simulink model "VdP_RCAC_ESC_sim"  (R2023b)
settings: Solver=ode4  StartTime=0.0  StopTime=Tf  FixedStep=Ts  RelTol=1e-3
values from neighbouring files (symbols this model uses):
  T_samp = 10    [VdP_RCAC_ESC.m]
  t_start = 20    [VdP_CL.m]    (also in VdP_RCAC_ESC.m)
  Ts = 0.001    [VdP_CL.m]    (also in VdP_RCAC_ESC.m)
  x0 = [1;0]    [VdP_CL.m]    (also in VdP_RCAC_ESC.m)
libraries: dspstat3 x1, matrix_library x1
settings Model: Creator=Juan Augusto Paredes  LastModifiedBy=Juan Augusto Paredes

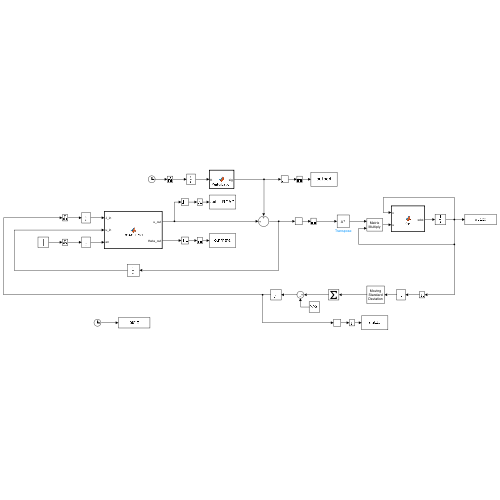
[thumbnail: Simulink's stored preview of the top-level diagram]
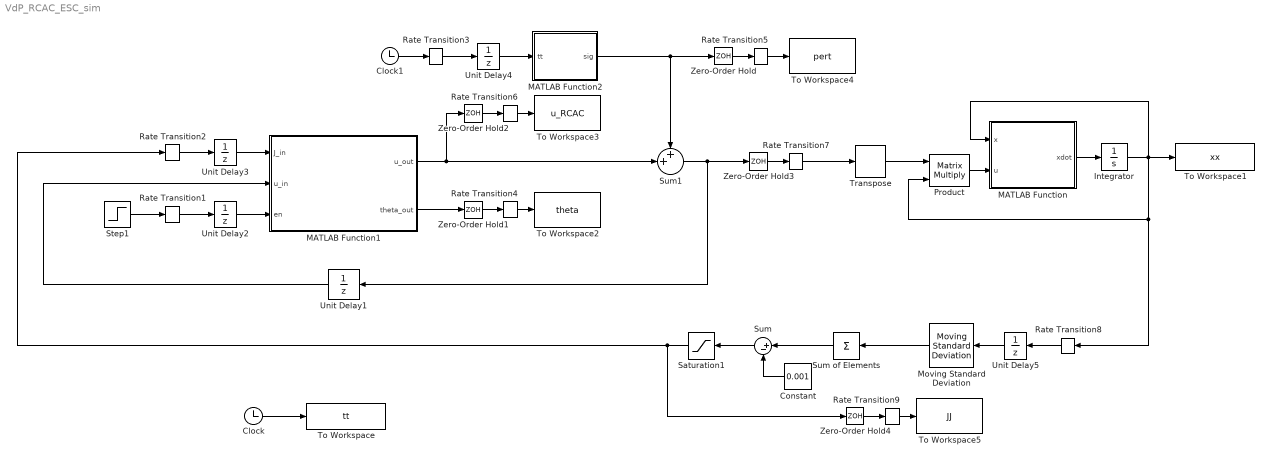
== system VdP_RCAC_ESC_sim ==
  Clock : Clock
  Clock1 : Clock
  Constant : Constant  Value=0.001
  Integrator : Integrator  InitialCondition=x0
  MATLAB Function : MATLAB Function  TreatAsAtomicUnit=on
  MATLAB Function1 : MATLAB Function  TreatAsAtomicUnit=on
  MATLAB Function2 : MATLAB Function  TreatAsAtomicUnit=on
  Moving Standard Deviation : dspstat3/Moving Standard Deviation  Method=Sliding window  ForgettingFactorPort=off  SpecifyWindowLength=on  WindowLength=5000  OverlapLength=4999  AllowArbitraryInputLength=off  ForgettingFactor=0.9  SimulateUsing=Code generation
  Product : Product  Multiplication=Matrix(*)
  Rate Transition{1..4,8..9} (6 alike) : RateTransition
  Rate Transition5 : RateTransition  InitialCondition=[0;0]
  Rate Transition6 : RateTransition  InitialCondition=[0;0]
  Rate Transition7 : RateTransition  InitialCondition=[0;0]
  Saturation1 : Saturate  UpperLimit=1000  LowerLimit=0
  Step1 : Step  Time=t_start  SampleTime=0
  Sum : Sum  Inputs=|+-
  Sum of Elements : Sum  Inputs=+
  Sum1 : Sum  Inputs=++|
  To Workspace : ToWorkspace  VariableName=tt  SampleTime=-1
  To Workspace1 : ToWorkspace  VariableName=xx  SampleTime=-1
  To Workspace2 : ToWorkspace  VariableName=theta  SampleTime=-1
  To Workspace3 : ToWorkspace  VariableName=u_RCAC  SampleTime=-1
  To Workspace4 : ToWorkspace  VariableName=pert  SampleTime=-1
  To Workspace5 : ToWorkspace  VariableName=JJ  SampleTime=-1
  Transpose : matrix_library/Transpose
  Unit Delay1 : UnitDelay  InitialCondition=[0;0]  SampleTime=T_samp  HasFrameUpgradeWarning=on
  Unit Delay2 : UnitDelay  SampleTime=T_samp  HasFrameUpgradeWarning=on
  Unit Delay3 : UnitDelay  SampleTime=T_samp  HasFrameUpgradeWarning=on
  Unit Delay4 : UnitDelay  SampleTime=T_samp  HasFrameUpgradeWarning=on
  Unit Delay5 : UnitDelay  SampleTime=Ts  HasFrameUpgradeWarning=on
  Zero-Order Hold{,1..4} (5 alike) : ZeroOrderHold  SampleTime=T_samp
  wires:
  MATLAB Function/1(xdot) -> Integrator/1
  Integrator/1 -> Rate Transition8/1, Product/2, To Workspace1/1, MATLAB Function/1(x)
  Clock/1 -> To Workspace/1
  Sum1/1 -> Zero-Order Hold3/1, Unit Delay1/1
  Unit Delay1/1 -> MATLAB Function1/2(u_in)
  MATLAB Function1/1(u_out) -> Zero-Order Hold2/1, Sum1/2
  Product/1 -> MATLAB Function/2(u)
  Transpose/1 -> Product/1
  Rate Transition1/1 -> Unit Delay2/1
  Unit Delay2/1 -> MATLAB Function1/3(en)
  Step1/1 -> Rate Transition1/1
  Unit Delay3/1 -> MATLAB Function1/1(J_in)
  Rate Transition2/1 -> Unit Delay3/1
  Rate Transition3/1 -> Unit Delay4/1
  Clock1/1 -> Rate Transition3/1
  Unit Delay4/1 -> MATLAB Function2/1(tt)
  Zero-Order Hold1/1 -> Rate Transition4/1
  Rate Transition4/1 -> To Workspace2/1
  MATLAB Function1/2(theta_out) -> Zero-Order Hold1/1
  MATLAB Function2/1(sig) -> Zero-Order Hold/1, Sum1/1
  Zero-Order Hold/1 -> Rate Transition5/1
  Rate Transition5/1 -> To Workspace4/1
  Zero-Order Hold2/1 -> Rate Transition6/1
  Rate Transition6/1 -> To Workspace3/1
  Zero-Order Hold3/1 -> Rate Transition7/1
  Rate Transition7/1 -> Transpose/1
  Moving Standard Deviation/1 -> Sum of Elements/1
  Rate Transition8/1 -> Unit Delay5/1
  Unit Delay5/1 -> Moving Standard Deviation/1
  Rate Transition9/1 -> To Workspace5/1
  Zero-Order Hold4/1 -> Rate Transition9/1
  Saturation1/1 -> Zero-Order Hold4/1, Rate Transition2/1
  Sum of Elements/1 -> Sum/1
  Sum/1 -> Saturation1/1
  Constant/1 -> Sum/2

== matlab function VdP_RCAC_ESC_sim/MATLAB Function1 ==
  settings: updateMethod=DISCRETE  sampleTime=T_samp
  data: J_in input size=1; u_out output size=2; u_in input size=2; en input size=1; theta_out output size=40; Nc parameter size=1
function [u_out, theta_out] = RCAC_ESC(J_in, u_in, en, Nc)

persistent Grad_Est DDRCAC_Cont uouttemp thetaouttemp opts Nf_prev

if isempty(uouttemp)
    opts = RCAC_ESC_KF_MISO_define_opts();
    Grad_Est = grad_est_KF(opts.lu, opts.lz, opts.indi, opts.P0_G, opts.Q, opts.R);
    DDRCAC_Cont = DDRCAC(opts.lu, opts.lz, opts.Nc, opts.P0_C, opts.Ru, opts.nu);
    uouttemp = [0;0];
    thetaouttemp = zeros(4*Nc,1); 
    Nf_prev = [0 0];
end

theta_out = zeros(40,1); %Due to Max number for Nc = 10, can adjust by changing theta_out size

if en > 0.5
    %% Gradient estimation
    [Grad_Est, grad] = Grad_Est.oneStep(u_in, J_in, en);
    
    %% Gradient to Nf (MIMO)
    grad = grad.';
    gradNorm = sqrt(sum(grad.^2,2));
    gradNorm(gradNorm<=opts.epsi) = opts.epsi;
    % if gradNorm >= opts.epsi
         Nf_temp = grad./gradNorm;
    %     Nf_prev = Nf_temp;
    % else
    %     Nf_temp = Nf_prev;
    % end
    Nf = zeros(opts.lz,opts.lu*opts.lu);
    for ii = 1:opts.lu
        Nf(:,1+(ii-1)*(opts.lu+1)) = Nf_temp(:,ii);
    end
    
    %% RCAC with Nf (DDRCAC)
    [DDRCAC_Cont, uouttemp, thetaouttemp] = DDRCAC_Cont.oneStep(u_in, J_in, Nf, 0);

end

u_out = uouttemp(1:2,1);
theta_out(1:4*Nc,1) = thetaouttemp(1:4*Nc,1);

end

== matlab function VdP_RCAC_ESC_sim/MATLAB Function ==
  data: x input size=2; u input size=1; xdot output size=2
function xdot = fcn(x,u)

xdot = [x(2) ;...
        -x(1) - ((x(2))^2 - 1)*x(2) + u];

end

== matlab function VdP_RCAC_ESC_sim/MATLAB Function2 ==
  settings: updateMethod=DISCRETE  sampleTime=T_samp
  data: tt input size=1; sig output size=2; T_samp parameter size=1; t_start parameter size=1
function sig = Perturbation(tt,T_samp, t_start)
    sig = PertFcnMISOVdP(tt, T_samp, t_start);
end
